simulink model "histogram_AXIS_TMI_4pix"  (R2015b)
settings: Solver=FixedStepDiscrete  SolverMode=SingleTasking  StartTime=0.0  StopTime=StartTime  FixedStep=1  RelTol=1e-3
values from neighbouring files (symbols this model uses):
  Nb_bin = 128    [Histogram_aldec_validation.m]    (also in Histogram_init.m = 1024; Histogram_init_20163.m; Histogram_init_validation.m)
  Ts = 1    [Histogram_aldec_validation.m]    (also in Histogram_init.m; Histogram_init_20163.m; Histogram_init_validation.m)
libraries: xbsIndex_r4 x172
(part 2 of 2)

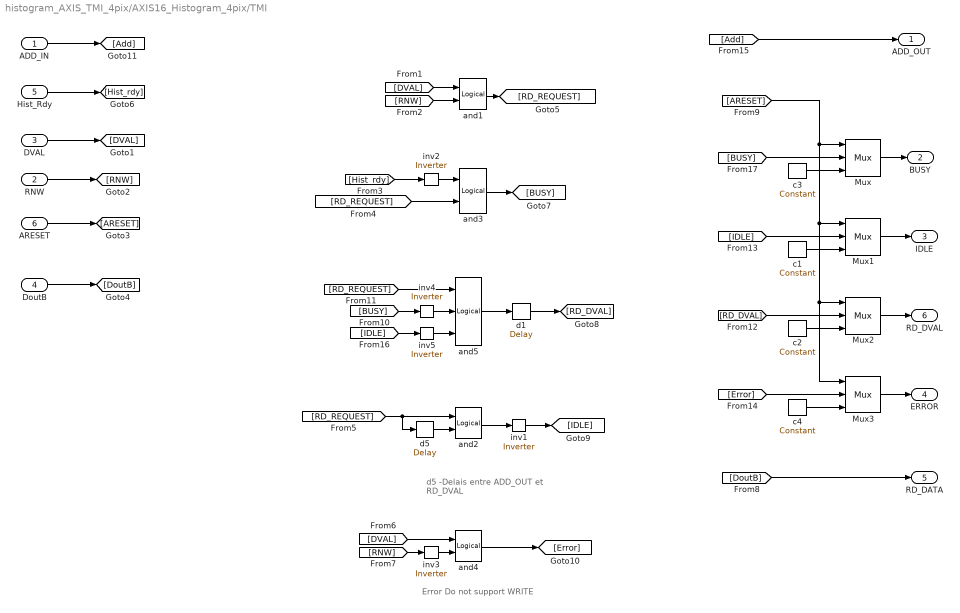
== system histogram_AXIS_TMI_4pix/AXIS16_Histogram_4pix/TMI ==
  note: d5 -Delais entre ADD_OUT
      |  et RD_DVAL
  note: Error Do not support WRITE
  ADD_IN : Inport
  RNW : Inport  Port=2
  DVAL : Inport  Port=3
  DoutB : Inport  Port=4
  Hist_Rdy : Inport  Port=5
  ARESET : Inport  Port=6
  Mux{,1..3} (4 alike) : xbsIndex_r4/Mux  inputs=2  en=off  latency=0  precision=Full  arith_type=Unsigned  n_bits=16  bin_pt=14  quantization=Truncate  overflow=Wrap  dbl_ovrd=off  block_type=mux
      settings: xl_area=[1 0 0 1 0 0 0]
  and1 : xbsIndex_r4/Logical  logical_function=AND  inputs=2  en=off  latency=0  precision=Full  arith_type=Unsigned  n_bits=16  bin_pt=0  align_bp=on  dbl_ovrd=off  block_type=logical
      settings: xl_area=[1 0 0 1 0 0 0]
  and2 : xbsIndex_r4/Logical  logical_function=OR  inputs=2  en=off  latency=0  precision=Full  arith_type=Unsigned  n_bits=16  bin_pt=0  align_bp=on  dbl_ovrd=off  block_type=logical
      settings: xl_area=[1 0 0 1 0 0 0]
  and3 : xbsIndex_r4/Logical  logical_function=AND  inputs=2  en=off  latency=0  precision=Full  arith_type=Unsigned  n_bits=16  bin_pt=0  align_bp=on  dbl_ovrd=off  block_type=logical
      settings: xl_area=[1 0 0 1 0 0 0]
  and4 : xbsIndex_r4/Logical  logical_function=AND  inputs=2  en=off  latency=0  precision=Full  arith_type=Unsigned  n_bits=16  bin_pt=0  align_bp=on  dbl_ovrd=off  block_type=logical
      settings: xl_area=[1 0 0 1 0 0 0]
  and5 : xbsIndex_r4/Logical  logical_function=AND  inputs=3  en=off  latency=0  precision=Full  arith_type=Unsigned  n_bits=16  bin_pt=0  align_bp=on  dbl_ovrd=off  block_type=logical
      settings: xl_area=[1 0 0 1 0 0 0]
  c1 : xbsIndex_r4/Constant  const=0  gui_display_data_type=Boolean  arith_type=Boolean  n_bits=MaxHistValue_bit  bin_pt=0  preci_type=Single  exp_width=8  frac_width=24  explicit_period=off  period=1  equ=P=C  opselect=C  inp2=PCIN>>17  opr=+  inp1=P  carry=CIN  dbl_ovrd=off  block_type=constant
  c2 : xbsIndex_r4/Constant  const=0  gui_display_data_type=Boolean  arith_type=Boolean  n_bits=MaxHistValue_bit  bin_pt=0  preci_type=Single  exp_width=8  frac_width=24  explicit_period=off  period=1  equ=P=C  opselect=C  inp2=PCIN>>17  opr=+  inp1=P  carry=CIN  dbl_ovrd=off  block_type=constant
  c3 : xbsIndex_r4/Constant  const=1  gui_display_data_type=Boolean  arith_type=Boolean  n_bits=MaxHistValue_bit  bin_pt=0  preci_type=Single  exp_width=8  frac_width=24  explicit_period=off  period=1  equ=P=C  opselect=C  inp2=PCIN>>17  opr=+  inp1=P  carry=CIN  dbl_ovrd=off  block_type=constant
  c4 : xbsIndex_r4/Constant  const=0  gui_display_data_type=Boolean  arith_type=Boolean  n_bits=MaxHistValue_bit  bin_pt=0  preci_type=Single  exp_width=8  frac_width=24  explicit_period=off  period=1  equ=P=C  opselect=C  inp2=PCIN>>17  opr=+  inp1=P  carry=CIN  dbl_ovrd=off  block_type=constant
  d1 : xbsIndex_r4/Delay  rst=off  infoeditControl=Selection of Reset will increase slice count due to use of real FFs and instead of SRLs  en=off  latency=1  reg_retiming=off  dbl_ovrd=off  block_type=delay
      settings: xl_area=[1 1 0 0 0 0 0]
  d5 : xbsIndex_r4/Delay  rst=off  infoeditControl=Selection of Reset will increase slice count due to use of real FFs and instead of SRLs  en=off  latency=1  reg_retiming=off  dbl_ovrd=off  block_type=delay
      settings: xl_area=[1 1 0 0 0 0 0]
  inv{1..5} (5 alike) : xbsIndex_r4/Inverter  en=off  latency=0  dbl_ovrd=off  block_type=inv
      settings: xl_area=[0 0 0 0 0 0 0]
  ADD_OUT : Outport
  BUSY : Outport  Port=2
  IDLE : Outport  Port=3
  ERROR : Outport  Port=4
  RD_DATA : Outport  Port=5
  RD_DVAL : Outport  Port=6
  wires:
  Hist_Rdy/1 -> [Hist_rdy]
  DVAL/1 -> [DVAL]
  RNW/1 -> [RNW]
  ARESET/1 -> [ARESET]
  DoutB/1 -> [DoutB]
  [DVAL] -> and1/1
  [RNW] -> and1/2
  d5/1 -> and2/2
  and2/1 -> inv1/1
  inv2/1 -> and3/1
  [Hist_rdy] -> inv2/1
  [RD_REQUEST] -> and3/2
  and1/1 -> [RD_REQUEST]
  [RD_REQUEST] -> and2/1, d5/1
  [DVAL] -> and4/1
  [RNW] -> inv3/1
  inv3/1 -> and4/2
  [DoutB] -> RD_DATA/1
  and3/1 -> [BUSY]
  [BUSY] -> inv4/1
  and5/1 -> d1/1
  d1/1 -> [RD_DVAL]
  inv1/1 -> [IDLE]
  and4/1 -> [Error]
  ADD_IN/1 -> [Add]
  [Add] -> ADD_OUT/1
  inv5/1 -> and5/3
  [IDLE] -> inv5/1
  Mux/1 -> BUSY/1
  [ARESET] -> Mux/1, Mux1/1, Mux2/1, Mux3/1
  [BUSY] -> Mux/2
  c3/1 -> Mux/3
  Mux1/1 -> IDLE/1
  [IDLE] -> Mux1/2
  c1/1 -> Mux1/3
  Mux2/1 -> RD_DVAL/1
  [RD_DVAL] -> Mux2/2
  c2/1 -> Mux2/3
  Mux3/1 -> ERROR/1
  [Error] -> Mux3/2
  c4/1 -> Mux3/3
  [RD_REQUEST] -> and5/1
  inv4/1 -> and5/2

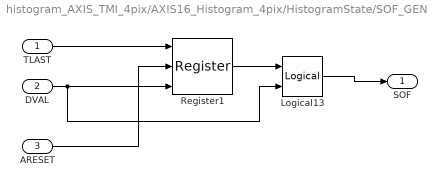
== system histogram_AXIS_TMI_4pix/AXIS16_Histogram_4pix/HistogramState/SOF_GEN ==
  TLAST : Inport
  DVAL : Inport  Port=2
  "ARESET " : Inport  Port=3
  Logical13 : xbsIndex_r4/Logical  logical_function=AND  inputs=2  en=off  latency=0  precision=Full  arith_type=Unsigned  n_bits=16  bin_pt=0  align_bp=on  dbl_ovrd=off  block_type=logical
      settings: xl_area=[1 0 0 1 0 0 0]
  Register1 : xbsIndex_r4/Register  init=1  rst=on  en=on  dbl_ovrd=off  block_type=register
  SOF : Outport
  wires:
  TLAST/1 -> Register1/1
  Register1/1 -> Logical13/1
  DVAL/1 -> Logical13/2, Register1/3
  Logical13/1 -> SOF/1
  "ARESET "/1 -> Register1/2
